simulink model "ECE411_prj_LockedRotorStepResponse12"  (R2023b)
settings: Solver=VariableStepAuto  StartTime=0.0  StopTime=0.2  RelTol=1e-3
values from neighbouring files (symbols this model uses):
  P = 8    [ECE411_HW2_2_Parameters.m]    (also in main_code.m)
  Vstep = 1.0    (= 1)    [ECE411_HW2_2_Parameters.m]    (also in main_code.m)
libraries: fl_lib x12, nesl_utility x11, ee_lib x1
settings Model: Creator=DiggerPC  LastModifiedBy=baik3-ad
settings DebuggingCC: UnconnectedInputMsg=warning  UnconnectedOutputMsg=warning  UnconnectedLineMsg=warning
settings ModelReferenceCC: EnableRefExpFcnMdlSchedulingChecks=on
settings RTWCC: DLArmComputeVersion=19.05

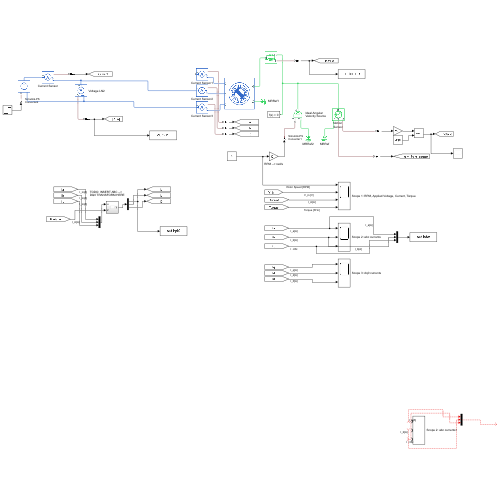
[thumbnail: Simulink's stored preview of the top-level diagram]
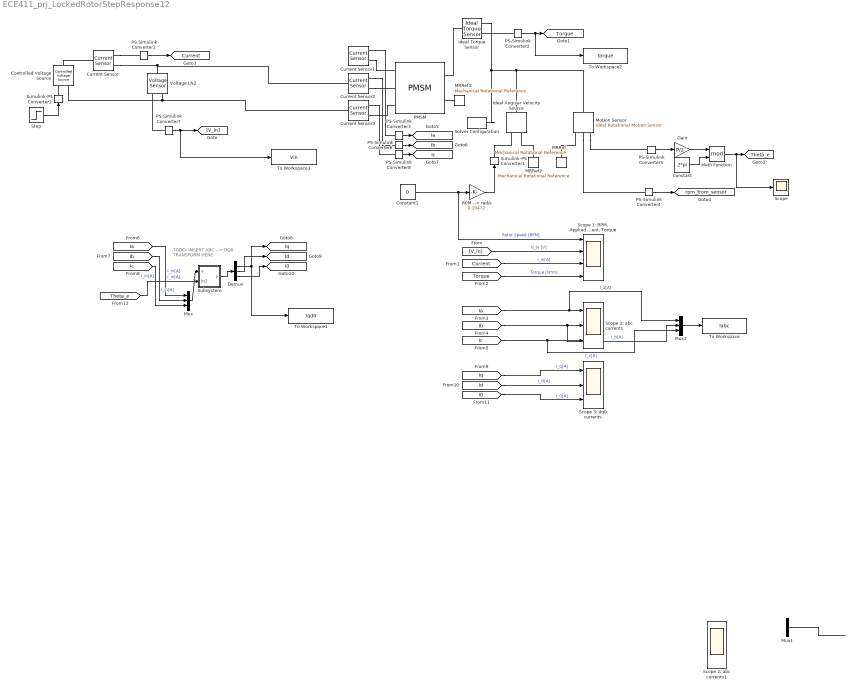
== system ECE411_prj_LockedRotorStepResponse12 ==
  note: TODO: INSERT ABC --> DQ0 TRANSFORM HERE
  Constant : Constant  Value=2*pi
  Constant1 : Constant  Value=0
  Controlled Voltage Source : fl_lib/Electrical/Electrical Sources/Controlled Voltage Source
  Current Sensor{,1..3} (4 alike) : fl_lib/Electrical/Electrical Sensors/Current Sensor
  Demux : Demux  Outputs=3
  Gain : Gain  Gain=P/2
  Ideal Angular Velocity Source : fl_lib/Mechanical/Mechanical Sources/Ideal Angular Velocity Source
  Ideal Torque Sensor : fl_lib/Mechanical/Mechanical Sensors/Ideal Torque Sensor
  MRRef : fl_lib/Mechanical/Rotational Elements/Mechanical Rotational Reference
  MRRef1 : fl_lib/Mechanical/Rotational Elements/Mechanical Rotational Reference
  MRRef2 : fl_lib/Mechanical/Rotational Elements/Mechanical Rotational Reference
  Math Function : Math  Operator=mod
  Motion Sensor : fl_lib/Mechanical/Mechanical Sensors/Ideal Rotational Motion Sensor  reference=foundation.enum.MeasurementReference.difference  acceleration_port=false  velocity_port=true  position_port=true  wrap_angle=simscape.enum.onoff.on  offset=0 deg
  Mux : Mux  Inputs=3
  Mux1 : Mux  Inputs=3
  Mux2 : Mux  Inputs=3
  PMSM : ee_lib/Electromechanical/Permanent Magnet/PMSM  port_option=ee.enum.threePhasePort.expanded  winding_type=ee.enum.statorconnection.wye  machine_param=ee.enum.pmsm.parameterization.constant  nPolePairs=P/2  pmflux_param=ee.enum.pmflux.fluxlinkage  pm_flux_linkage=lambda_f Wb  torque_constant=0.037*sqrt(2) N*m/A  back_emf_constant=0.037*sqrt(2) V/(rad/s)  stator_param=ee.enum.statorparam.LdLqL0  Ld=Lq H  Lq=Ld H  idVec=[-200, 0, 200] A  iqVec=[-200, 0, 200] A  LdMatrix=0.0002 * ones(3, 3) H  LqMatrix=0.0002 * ones(3, 3) H  PmMatrix=0.1 * ones(3, 3) Wb  ktMatrix=0.18 * ones(3, 3) N*m/A  keMatrix=0.18 * ones(3, 3) V/(rad/s)  L0=L0 H  Ls=Ls H  Lm=0 H  Ms=0 H  Rs=Rs Ohm  zero_sequence=ee.enum.park.zerosequence.exclude  axes_param=ee.enum.rotorangle.qaxis  loss_param=ee.enum.ironloss.none  losses_oc=[0, 0, 0] W  losses_sc=[0, 0, 0] W  f_losses=60 Hz  Isc_losses=95 A  J=0.01 kg*m^2  lam=0 N*m/(rad/s)  i_d_specify=off  i_d_priority=None  i_d=0 A  i_d_nominal_specify=off  i_d_nominal_unit=A  i_d_nominal_value=1  i_q_specify=off  i_q_priority=None  i_q=0 A  i_q_nominal_specify=off  i_q_nominal_unit=A  i_q_nominal_value=1  torque_specify=off  torque_priority=None  torque=0 N*m  torque_nominal_specify=off  torque_nominal_unit=N*m  torque_nominal_value=1  angular_velocity_specify=off  angular_velocity_priority=High  angular_velocity=0 rpm  angular_velocity_nominal_specify=off  angular_velocity_nominal_unit=rpm  angular_velocity_nominal_value=1  angular_position_specify=off  angular_position_priority=High  angular_position=0 deg  angular_position_nominal_specify=off  angular_position_nominal_unit=deg  angular_position_nominal_value=1  alpha=3.93e-3 1/K  alpha_flux=-0.001 1/K  Tmeas=298.15 K  stator_thermal_mass=100 J/K  rotor_thermal_mass=200 J/K  Rm_percent_rotor=90  Rd_percent_rotor=30  temperatureA_specify=off  temperatureA_priority=High  temperatureA=25 degC  temperatureA_nominal_specify=off  temperatureA_nominal_unit=degC  temperatureA_nominal_value=1  temperatureB_specify=off  temperatureB_priority=High  temperatureB=25 degC  temperatureB_nominal_specify=off  temperatureB_nominal_unit=degC  temperatureB_nominal_value=1  temperatureC_specify=off  temperatureC_priority=High  temperatureC=25 degC  temperatureC_nominal_specify=off  temperatureC_nominal_unit=degC  temperatureC_nominal_value=1  temperatureR_specify=off  temperatureR_priority=High  temperatureR=25 degC  temperatureR_nominal_specify=off  temperatureR_nominal_unit=degC  temperatureR_nominal_value=1
      settings: InternalSimscapePortConfiguration="{\"Bottom\":[],\"Left\":[{\"id\":\"a\",\"label\":\"a\",\"type\":\"foundation.electrical.electrical\"},{\"id\":\"b\",\"label\":\"b\",\"type\":\"foundation.electrical.electrical\"},{\"id\":\"c\",\"label\":\"c\",\"type\":\"foundation.electrical.electrical\"}],\"Right\":[{\"id\":\"R\",\"label\":\"R\",\"type\":\"foundation.mechanical.rotational.rotational\"},{\"id\":\"C\",\"label\":\"C\",\"type\":\"foundation.mechanical.rotational.rotational\"}],\"Top\":[]}"
  PS-Simulink Converter{1,3,6,8} (4 alike) : nesl_utility/PS-Simulink Converter  PhysicalDomain=network_engine_domain  SubClassName=ps_output  LeftPortType=input  RightPortType=output  PseudoPeriodic=off  Frequencies=[]  VectorFormat=1-D array  Unit=A  AffineConversion=off
  PS-Simulink Converter2 : nesl_utility/PS-Simulink Converter  PhysicalDomain=network_engine_domain  SubClassName=ps_output  LeftPortType=input  RightPortType=output  PseudoPeriodic=off  Frequencies=[]  VectorFormat=1-D array  Unit=N*m  AffineConversion=off
  PS-Simulink Converter4 : nesl_utility/PS-Simulink Converter  PhysicalDomain=network_engine_domain  SubClassName=ps_output  LeftPortType=input  RightPortType=output  PseudoPeriodic=off  Frequencies=[]  VectorFormat=1-D array  Unit=rpm  AffineConversion=off
  PS-Simulink Converter5 : nesl_utility/PS-Simulink Converter  PhysicalDomain=network_engine_domain  SubClassName=ps_output  LeftPortType=input  RightPortType=output  PseudoPeriodic=off  Frequencies=[]  VectorFormat=1-D array  Unit=rad  AffineConversion=off
  PS-Simulink Converter7 : nesl_utility/PS-Simulink Converter  PhysicalDomain=network_engine_domain  SubClassName=ps_output  LeftPortType=input  RightPortType=output  PseudoPeriodic=off  Frequencies=[]  VectorFormat=1-D array  Unit=V  AffineConversion=off
  RPM --> rad/s : Gain  Gain=0.10472
  Scope : Scope
  "Scope 1: RPM, Applied Voltage, Current, Torque" : Scope  NumInputPorts=4
  Scope 2: abc currents : Scope  NumInputPorts=3
  Scope 2: abc currents1 : Scope  NumInputPorts=3
  Scope 3: dq0 currents : Scope  NumInputPorts=3
  Simulink-PS Converter1 : nesl_utility/Simulink-PS Converter  PhysicalDomain=network_engine_domain  SubClassName=ps_input  LeftPortType=input  RightPortType=output  PseudoPeriodic=off  Frequencies=[]  NoiseDistribution=none  NoiseParameters=[]  Unit=rad/s  AffineConversion=off  FilteringAndDerivatives=zero  SimscapeFilterOrder=1  InputFilterTimeConstant=0.001  UdotUserProvided=1
  Simulink-PS Converter2 : nesl_utility/Simulink-PS Converter  PhysicalDomain=network_engine_domain  SubClassName=ps_input  LeftPortType=input  RightPortType=output  PseudoPeriodic=off  Frequencies=[]  NoiseDistribution=none  NoiseParameters=[]  Unit=V  AffineConversion=off  FilteringAndDerivatives=zero  SimscapeFilterOrder=1  InputFilterTimeConstant=0.001  UdotUserProvided=1
  Solver Configuration : nesl_utility/Solver Configuration  PhysicalDomain=network_engine_domain  SubClassName=solver  LeftPortType=input  RightPortType=generic  Tones=[]  Harmonics=[]  SimulateNoise=off  Profile=off  UseLocalSampling=off  EnableSwitchedLinearOptims=on  FrequencyDomain=off  UseCCode=off  RelTol=0.001  AbsTol=1e-06  MinStep=1e-09  ToWorkspace=off  RevertToSquareIcSolve=off  NumHomotopyIterations=100  PhasorMode=off  PhasorModeNumHarmonics=1  ConsistencySolver=NEWTON_FTOL  IndexReductionMethod=DerivativeReplacement  DoDC=off  ResidualTolerance=1e-09  ConsistencyTolSource=GLOBAL  ConsistencyAbsTol=0.001  ConsistencyRelTol=0.001  ConsistencyTolFactor=0.001  UseLocalSolver=on  LocalSolverChoice=NE_TRAPEZOIDAL_ADVANCER  ResolveIndetEquations=on  FunctionEvalNumThread=1  LocalSolverSampleTime=1e-6  DoFixedCost=on  MaxNonlinIter=3  MaxModeIter=2  ComputeImpulses=off  ImpulseIterations=2  LinearAlgebra=auto  LinearAlgebraNumThread=0  EquationFormulation=NE_TIME_EF  DelaysMemoryBudget=1024  AutomaticFiltering=on  FilteringTimeConstant=0.001  PartitionStorageMethod=AS_NEEDED  PartitionMemoryBudget=1024  PartitionMethod=ROBUST  MultibodyUseLocalSolver=off  MultibodyLocalSolverChoice=ODE1  MultibodyLocalSolverSampleTime=0.001
  Step : Step  Time=0.1  After=Vstep  SampleTime=0
  Subsystem : Subsystem
  To Workspace : ToWorkspace  VariableName=Iabc  SaveFormat=Timeseries  SampleTime=-1
  To Workspace1 : ToWorkspace  VariableName=Iqd0  SaveFormat=Timeseries  SampleTime=-1
  To Workspace2 : ToWorkspace  VariableName=torque  SaveFormat=Timeseries  SampleTime=-1
  To Workspace3 : ToWorkspace  VariableName=Vin  SaveFormat=Timeseries  SampleTime=-1
  Voltage LN2 : fl_lib/Electrical/Electrical Sensors/Voltage Sensor
  tag scope: Current=global, I0=global, Ia=global, Ib=global, Ic=global, Id=global, Iq=global, Theta_e=global, Torque=global, rpm_from_sensor=global
  wires:
  RPM --> rad/s/1 -> Simulink-PS Converter1/1
  PS-Simulink Converter4/1 -> [rpm_from_sensor]
  Constant1/1 -> RPM --> rad/s/1, "Scope 1: RPM, Applied Voltage, Current, Torque"/1  "Rotor Speed [RPM]"
  PS-Simulink Converter5/1 -> Gain/1
  [Current] -> "Scope 1: RPM, Applied Voltage, Current, Torque"/3  "I_in[A]"
  Gain/1 -> Math Function/1
  [V_in] -> "Scope 1: RPM, Applied Voltage, Current, Torque"/2  "V_in [V]"
  [Torque] -> "Scope 1: RPM, Applied Voltage, Current, Torque"/4  "Torque [N*m]"
  Math Function/1 -> Scope/1, [Theta_e]
  Constant/1 -> Math Function/2
  PS-Simulink Converter2/1 -> To Workspace2/1, [Torque]
  Step/1 -> Simulink-PS Converter2/1
  PS-Simulink Converter1/1 -> [Current]
  PS-Simulink Converter8/1 -> [Ic]
  PS-Simulink Converter6/1 -> [Ib]
  PS-Simulink Converter3/1 -> [Ia]
  Demux/2 -> [Id]
  Demux/3 -> [I0]
  Demux/1 -> [Iq], To Workspace1/1
  [Iq] -> Scope 3: dq0 currents/1  "I_q[A]"
  [Id] -> Scope 3: dq0 currents/2  "I_d[A]"
  [I0] -> Scope 3: dq0 currents/3  "I_0[A]"
  [Ia] -> Mux2/1, Scope 2: abc currents/1  "I_a[A]"
  [Ib] -> Mux2/2, Scope 2: abc currents/2  "I_b[A]"
  [Ic] -> Mux2/3, Scope 2: abc currents/3  "I_c[A]"
  [Ia] -> Mux/1  "I_in[A]"
  Mux/1 -> Subsystem/1(u)
  [Ib] -> Mux/2  "I_in[A]"
  [Ic] -> Mux/3  "I_in[A]"
  [Theta_e] -> Subsystem/2(In2)  "I_in[A]"
  Subsystem/1(y) -> Demux/1
  PS-Simulink Converter7/1 -> To Workspace3/1, [V_in]
  ? -> Mux1/3  "I_c[A]"
  Mux1/1 -> ?
  ? -> Mux1/1  "I_a[A]"
  ? -> Mux1/2  "I_b[A]"
  Mux2/1 -> To Workspace/1
  connections:
  Motion Sensor/LConn1 -- Ideal Angular Velocity Source/LConn1 -- Solver Configuration/RConn1 -- Ideal Torque Sensor/RConn1
  Simulink-PS Converter1/RConn1 -- Ideal Angular Velocity Source/RConn1
  Motion Sensor/RConn3 -- PS-Simulink Converter5/LConn1
  MRRef/LConn1 -- Motion Sensor/RConn1
  Motion Sensor/RConn2 -- PS-Simulink Converter4/LConn1
  MRRef2/LConn1 -- Ideal Angular Velocity Source/RConn2
  PMSM/RConn2 -- MRRef1/LConn1
  PS-Simulink Converter7/LConn1 -- Voltage LN2/RConn1
  Ideal Torque Sensor/LConn1 -- PMSM/RConn1
  PS-Simulink Converter2/LConn1 -- Ideal Torque Sensor/RConn2
  Current Sensor/LConn1 -- Controlled Voltage Source/LConn1
  Simulink-PS Converter2/RConn1 -- Controlled Voltage Source/RConn1
  Current Sensor/RConn1 -- PS-Simulink Converter1/LConn1
  Controlled Voltage Source/RConn2 -- Current Sensor3/LConn1 -- Voltage LN2/RConn2
  Current Sensor/RConn2 -- Current Sensor2/LConn1 -- Voltage LN2/LConn1
  Current Sensor1/RConn2 -- PMSM/LConn1
  Current Sensor2/RConn2 -- PMSM/LConn2
  PMSM/LConn3 -- Current Sensor3/RConn2
  Current Sensor1/RConn1 -- PS-Simulink Converter3/LConn1
  Current Sensor2/RConn1 -- PS-Simulink Converter6/LConn1
  Current Sensor3/RConn1 -- PS-Simulink Converter8/LConn1

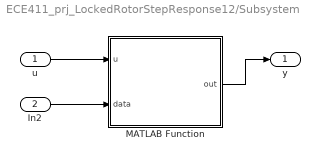
== system ECE411_prj_LockedRotorStepResponse12/Subsystem ==
  u : Inport
  In2 : Inport  Port=2
  MATLAB Function : MATLAB Function  TreatAsAtomicUnit=on
  y : Outport
  wires:
  u/1 -> MATLAB Function/1(u)
  In2/1 -> MATLAB Function/2(data)
  MATLAB Function/1(out) -> y/1

== matlab function ECE411_prj_LockedRotorStepResponse12/Subsystem/MATLAB Function ==
  data: u input; out output; data input
function out = fcn(u, data)

T1 = 2/3*[1 -1/2 -1/2;0 -sqrt(3)/2 sqrt(3)/2; 1/sqrt(2) 1/sqrt(2) 1/sqrt(2)];
alphabeta0= T1*u;

T2 = [cos(data) -sin(data) 0;sin(data) cos(data) 0; 0 0 1];
out = T2*alphabeta0;
end
